simulink model "shoukong"  (R2024b)
settings: Solver=VariableStepAuto  StartTime=0.0  StopTime=10.0  RelTol=1e-3
undefined symbols (not defined in the file): A, B, C, K, L, x_eq, y_eq
settings Model: Creator=54238  LastModifiedBy=54238

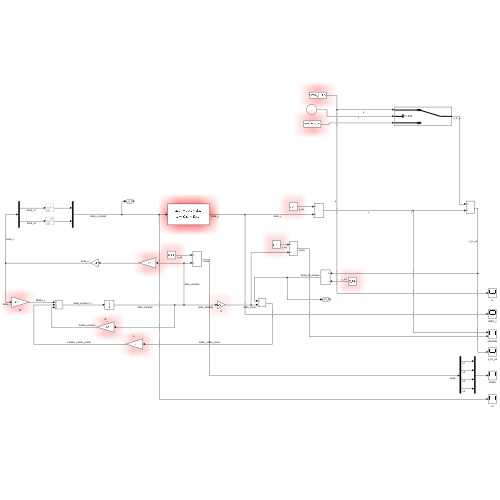
[thumbnail: Simulink's stored preview of the top-level diagram]
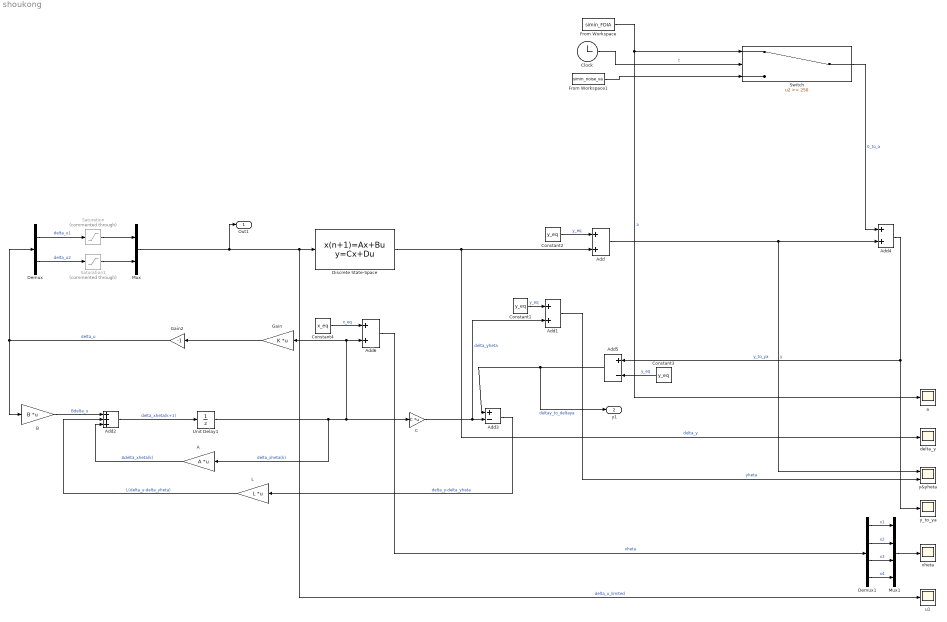
== system shoukong ==
  A : Gain  Gain=A  Multiplication=Matrix(K*u)
  Add{,1,4,6} (4 alike) : Sum
  Add2 : Sum  Inputs=+++
  Add3 : Sum  Inputs=+-
  Add5 : Sum  Inputs=+-
  B : Gain  Gain=B  Multiplication=Matrix(K*u)
  C : Gain  Gain=C  Multiplication=Matrix(K*u)
  Clock : Clock
  Constant1 : Constant  Value=y_eq  VectorParams1D=off
  Constant2 : Constant  Value=y_eq  VectorParams1D=off
  Constant3 : Constant  Value=y_eq  VectorParams1D=off
  Constant4 : Constant  Value=x_eq  VectorParams1D=off
  Demux : Demux  Outputs=2
  Demux1 : Demux
  Discrete State-Space : DiscreteStateSpace  A=A  B=B  C=C  D=[0 0;0 0]  InitialCondition=[0.5 0.5 0.1 0.1]  SampleTime=-1
  From Workspace : FromWorkspace  VariableName=simin_FDIA  SampleTime=-1
  From Workspace1 : FromWorkspace  VariableName=simin_noise_va  SampleTime=-1
  Gain : Gain  Gain=K  Multiplication=Matrix(K*u)
  Gain2 : Gain  Gain=-1
  L : Gain  Gain=L  Multiplication=Matrix(K*u)
  Mux : Mux  Inputs=2
  Mux1 : Mux
  Saturation : Saturate  Commented=through  UpperLimit=0.999  LowerLimit=-0.999
  Saturation1 : Saturate  Commented=through  UpperLimit=1.005  LowerLimit=-1.005
  Switch : Switch  Threshold=250  SaturateOnIntegerOverflow=off  InputSameDT=off
  Unit Delay1 : UnitDelay  SampleTime=-1  HasFrameUpgradeWarning=on
  a : Scope
  delta_y : Scope
  u1 : Scope
  xheta : Scope
  y&yheta : Scope  NumInputPorts=2
  y_to_ya : Scope
  Out1 : Outport  PortDimensions=[2,1]
  y1 : Outport  Port=2  PortDimensions=[2,1]
  wires:
  Mux/1 -> Out1/1, u1/1, Discrete State-Space/1  "delta_u_limited"
  B/1 -> Add2/1  "Bdelta_u"
  Constant2/1 -> Add/1  "y_eq"
  Switch/1 -> Add4/1  "0_to_a"
  Demux1/3 -> Mux1/3  "x3"
  Constant4/1 -> Add6/1  "x_eq"
  Gain2/1 -> Demux/1, B/1  "delta_u"
  Demux/1 -> Saturation/1  "delta_u1"
  Gain/1 -> Gain2/1
  Add/1 -> y&yheta/1, Add4/2  "y"
  From Workspace/1 -> Switch/1, a/1  "a"
  Demux1/2 -> Mux1/2  "x2"
  Demux1/4 -> Mux1/4  "x4"
  Add6/1 -> Demux1/1  "xheta"
  Demux/2 -> Saturation1/1  "delta_u2"
  Add5/1 -> y1/1, Add3/1  "deltay_to_deltaya"
  From Workspace1/1 -> Switch/3
  Add1/1 -> y&yheta/2  "yheta"
  Add4/1 -> Add5/1, y_to_ya/1  "y_to_ya"
  Discrete State-Space/1 -> delta_y/1, Add/2  "delta_y"
  A/1 -> Add2/3  "Adelta_xheta(k)"
  Unit Delay1/1 -> Add6/2, Gain/1, C/1, A/1  "delta_xheta(k)"
  Saturation/1 -> Mux/1
  Add2/1 -> Unit Delay1/1  "delta_xheta(k+1)"
  Constant3/1 -> Add5/2  "y_eq"
  L/1 -> Add2/2  "L(delta_y-delta_yheta)"
  Mux1/1 -> xheta/1
  Saturation1/1 -> Mux/2
  C/1 -> Add1/2, Add3/2  "delta_yheta"
  Add3/1 -> L/1  "delta_y-delta_yheta"
  Clock/1 -> Switch/2  "t"
  Demux1/1 -> Mux1/1  "x1"
  Constant1/1 -> Add1/1  "y_eq"
